simulink model "PIDcontinuos_01"  (R2015a)
settings: Solver=ode3  StartTime=0.0  StopTime=10.0  FixedStep=0.1  RelTol=1e-3
values from neighbouring files (symbols this model uses):
  K = (y_real(end) - y_real(1))/(input.signals.values(end) - 0)    [ctr.m]
  kd_CC = kp_CC*td_CC    [ctr.m]
  kd_ZN = kp_ZN*td_ZN    [ctr.m]
  ki_CC = kp_CC/ti_CC    [ctr.m]
  ki_ZN = kp_ZN/ti_ZN    [ctr.m]
  kp_CC = T/(L*(4/3 + R/4))    [ctr.m]
  kp_ZN = 1.2*T/L    [ctr.m]
  L = 1.5*(t1_28 - (t2_63/3))    [ctr.m]
  T = 1.5*(t2_63 - t1_28)    [ctr.m]
settings Model: Creator=guima  LastModifiedBy=guima

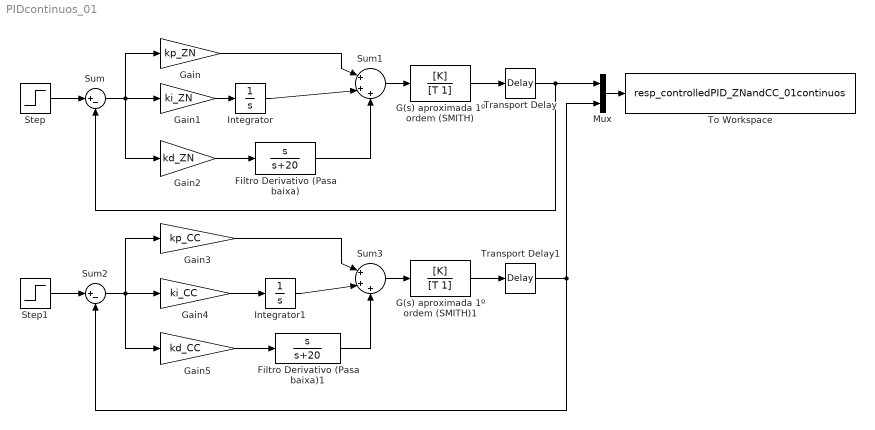
== system PIDcontinuos_01 ==
  Filtro Derivativo (Pasa baixa) : TransferFcn  Numerator=[1 0]  Denominator=[1 20]
  Filtro Derivativo (Pasa baixa)1 : TransferFcn  Numerator=[1 0]  Denominator=[1 20]
  G(s) aproximada 1º ordem (SMITH) : TransferFcn  Numerator=[K]  Denominator=[T 1]
  G(s) aproximada 1º ordem (SMITH)1 : TransferFcn  Numerator=[K]  Denominator=[T 1]
  Gain : Gain  Gain=kp_ZN
  Gain1 : Gain  Gain=ki_ZN
  Gain2 : Gain  Gain=kd_ZN
  Gain3 : Gain  Gain=kp_CC
  Gain4 : Gain  Gain=ki_CC
  Gain5 : Gain  Gain=kd_CC
  Integrator : Integrator
  Integrator1 : Integrator
  Mux : Mux  Inputs=2
  Step : Step  Time=0  SampleTime=0
  Step1 : Step  Time=0  SampleTime=0
  Sum : Sum  Inputs=|+-
  Sum1 : Sum  Inputs=|+++
  Sum2 : Sum  Inputs=|+-
  Sum3 : Sum  Inputs=|+++
  To Workspace : ToWorkspace  VariableName=resp_controlledPID_ZNandCC_01continuos  SaveFormat=Structure With Time  SampleTime=-1
  Transport Delay : TransportDelay  DelayTime=L
  Transport Delay1 : TransportDelay  DelayTime=L
  wires:
  Step/1 -> Sum/1
  Gain1/1 -> Integrator/1
  Gain2/1 -> Filtro Derivativo (Pasa baixa)/1
  Gain/1 -> Sum1/1
  Integrator/1 -> Sum1/2
  Filtro Derivativo (Pasa baixa)/1 -> Sum1/3
  Sum/1 -> Gain2/1, Gain/1, Gain1/1
  Sum1/1 -> G(s) aproximada 1º ordem (SMITH)/1
  G(s) aproximada 1º ordem (SMITH)/1 -> Transport Delay/1
  Transport Delay/1 -> Mux/1, Sum/2
  Step1/1 -> Sum2/1
  Gain4/1 -> Integrator1/1
  Gain5/1 -> Filtro Derivativo (Pasa baixa)1/1
  Gain3/1 -> Sum3/1
  Integrator1/1 -> Sum3/2
  Filtro Derivativo (Pasa baixa)1/1 -> Sum3/3
  Sum2/1 -> Gain5/1, Gain3/1, Gain4/1
  Sum3/1 -> G(s) aproximada 1º ordem (SMITH)1/1
  G(s) aproximada 1º ordem (SMITH)1/1 -> Transport Delay1/1
  Transport Delay1/1 -> Mux/2, Sum2/2
  Mux/1 -> To Workspace/1
